simulink model "p2_hw6"  (R2022b)
settings: Solver=VariableStepAuto  StartTime=0.0  StopTime=10.0  RelTol=1e-3
settings Model: Creator=shivavafadar  LastModifiedBy=shivavafadar

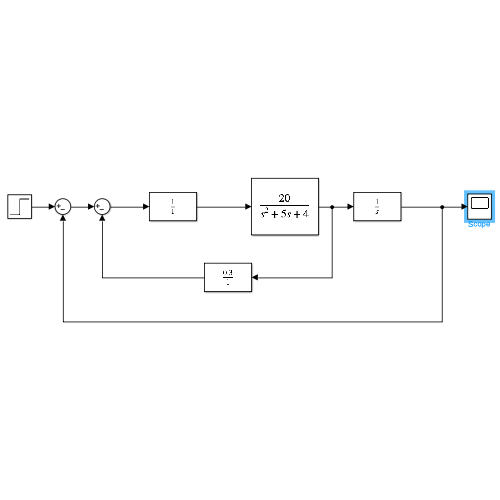
[thumbnail: Simulink's stored preview of the top-level diagram]
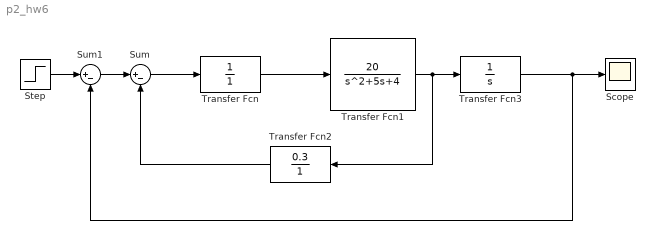
== system p2_hw6 ==
  Scope : Scope
  Step : Step  SampleTime=0
  Sum : Sum  Inputs=|+-
  Sum1 : Sum  Inputs=|+-
  Transfer Fcn : TransferFcn  Denominator=[ 1]
  Transfer Fcn1 : TransferFcn  Numerator=[20]  Denominator=[1 5 4]
  Transfer Fcn2 : TransferFcn  Numerator=[0.3]  Denominator=[ 1]
  Transfer Fcn3 : TransferFcn  Denominator=[1 0]
  wires:
  Transfer Fcn/1 -> Transfer Fcn1/1
  Transfer Fcn2/1 -> Sum/2
  Sum/1 -> Transfer Fcn/1
  Transfer Fcn1/1 -> Transfer Fcn2/1, Transfer Fcn3/1
  Sum1/1 -> Sum/1
  Transfer Fcn3/1 -> Scope/1, Sum1/2
  Step/1 -> Sum1/1
